simulink model "LeftSteeringWheelButtonsMgr"  (R2022b)
settings: configuration reference "CommonModelConfiguration" (kept outside this file)
undefined symbols (not defined in the file): cc_param_23, cc_param_36, LCFG_ButtonStuck, LCFG_HoldLong, LCFG_HoldShort
settings Model: Creator=sbaumga1  LastModifiedBy=othomso1
settings ConfigSetRef: SourceName=CommonModelConfiguration  SourceLocation=Base Workspace

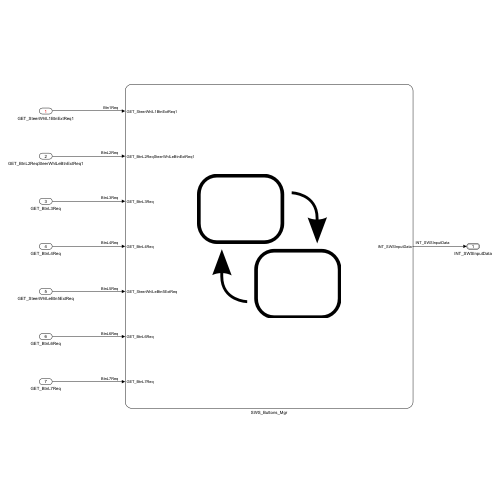
[thumbnail: Simulink's stored preview of the top-level diagram]
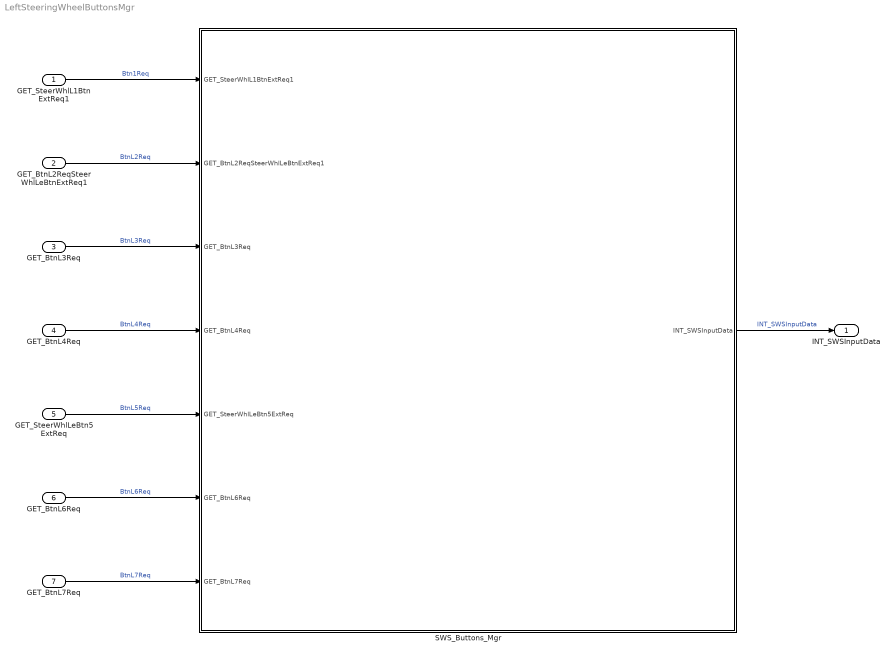
== system LeftSteeringWheelButtonsMgr ==
  GET_SteerWhlL1BtnExtReq1 : Inport  OutDataTypeStr=Enum: PsdNotPsd
  GET_BtnL2ReqSteerWhlLeBtnExtReq1 : Inport  Port=2  OutDataTypeStr=Enum: PsdNotPsd
  GET_BtnL3Req : Inport  Port=3  OutDataTypeStr=Enum: PsdNotPsd
  GET_BtnL4Req : Inport  Port=4  OutDataTypeStr=Enum: PsdNotPsd
  GET_SteerWhlLeBtn5ExtReq : Inport  Port=5  OutDataTypeStr=Enum: PsdNotPsd
  GET_BtnL6Req : Inport  Port=6  OutDataTypeStr=Enum: PsdNotPsd
  GET_BtnL7Req : Inport  Port=7  OutDataTypeStr=Enum: PsdNotPsd
  SWS_Buttons_Mgr : Stateflow chart  TreatAsAtomicUnit=on
  INT_SWSInputData : Outport  OutDataTypeStr=Bus: SWSInputData  BusOutputAsStruct=on
  wires:
  SWS_Buttons_Mgr/1(INT_SWSInputData) -> INT_SWSInputData/1  "INT_SWSInputData"
  GET_BtnL2ReqSteerWhlLeBtnExtReq1/1 -> SWS_Buttons_Mgr/2(GET_BtnL2ReqSteerWhlLeBtnExtReq1)  "BtnL2Req"
  GET_BtnL3Req/1 -> SWS_Buttons_Mgr/3(GET_BtnL3Req)  "BtnL3Req"
  GET_SteerWhlL1BtnExtReq1/1 -> SWS_Buttons_Mgr/1(GET_SteerWhlL1BtnExtReq1)  "Btn1Req"
  GET_BtnL4Req/1 -> SWS_Buttons_Mgr/4(GET_BtnL4Req)  "BtnL4Req"
  GET_SteerWhlLeBtn5ExtReq/1 -> SWS_Buttons_Mgr/5(GET_SteerWhlLeBtn5ExtReq)  "BtnL5Req"
  GET_BtnL6Req/1 -> SWS_Buttons_Mgr/6(GET_BtnL6Req)  "BtnL6Req"
  GET_BtnL7Req/1 -> SWS_Buttons_Mgr/7(GET_BtnL7Req)  "BtnL7Req"

== stateflow chart LeftSteeringWheelButtonsMgr/SWS_Buttons_Mgr ==
  state CARCONFIG_INVALID
  state SYSTEM_OK
    state sws = CheckPsdNotPsd [function]
      (default) -> (junction 458)
      (junction 458) -> (junction 459) [order 1] : [GET_SteerWhlL1BtnExtReq1 == PsdNotPsd.PsdNotPsd_Psd ||...
          | GET_BtnL2ReqSteerWhlLeBtnExtReq1 == PsdNotPsd.PsdNotPsd_Psd ||...
          | GET_BtnL3Req == PsdNotPsd.PsdNotPsd_Psd ||...
          | GET_BtnL4Req == PsdNotPsd.PsdNotPsd_Psd ||...
          | GET_SteerWhlLeBtn5ExtReq == PsdNotPsd.PsdNotPsd_Psd ||...
          | GET_BtnL6Req == PsdNotPsd.PsdNotPsd_Psd ||...
          | GET_BtnL7Req == PsdNotPsd.PsdNotPsd_Psd]
      (junction 458) -> (junction 384) [order 2] : {sws=false;}
      (junction 459) -> (junction 383) : {sws=true;}
      (junction 383) -> (junction 384)
      (junction 384) -> (junction 385)
    state IDLE
      en: INT_SWSInputData.Event = E_SWSEvent.Idle;
      release = false;
      ButtonsReset=false;
    state RELEASE
      en: INT_SWSInputData.Event = E_SWSEvent.Release;
    state PUSHED
      state RUNNING
        entry: ButtonPushed(); btnPush();
        during: ButtonPushed();
        state EVENT
          state PENDING
          state PENDING2
          state HOLDSHORT
            entry: INT_SWSInputData.Event = E_SWSEvent.HoldShort;
          state HOLDLONG
            entry: INT_SWSInputData.Event = E_SWSEvent.HoldLong;
          (default) -> (junction 299)
          (junction 299) -> (junction 488) [order 1] : [INT_SWSInputData.Button == E_SWSButton.BtnL4Req || INT_SWSInputData.Button == E_SWSButton.BtnL5Req]
              | {release = true;}
          (junction 299) -> PENDING [order 2]
          (junction 488) -> PENDING2
          PENDING2 -> HOLDSHORT : [after(LCFG_HoldShort, sec)]
          HOLDSHORT -> HOLDLONG : [after(LCFG_HoldLong, sec)]
        state INVALID_REQUEST
          state IDLE
            en: INT_SWSInputData.Event = E_SWSEvent.Idle;
          state DEACTIVATION
            en: INT_SWSInputData.Event = E_SWSEvent.Deactivation;
          (default) -> SYSTEM_OK.PUSHED.RUNNING.INVALID_REQUEST.IDLE
          SYSTEM_OK.PUSHED.RUNNING.INVALID_REQUEST.IDLE -> DEACTIVATION : [GET_SteerWhlL1BtnExtReq1==PsdNotPsd.PsdNotPsd_Psd]
          DEACTIVATION -> SYSTEM_OK.PUSHED.RUNNING.INVALID_REQUEST.IDLE : [GET_SteerWhlL1BtnExtReq1 ~= PsdNotPsd.PsdNotPsd_Psd]
        state btnPush [function]
          (default) -> (junction 9)
          (junction 9) -> (junction 15) [order 1] : [GET_SteerWhlL1BtnExtReq1 == PsdNotPsd.PsdNotPsd_Psd || GET_BtnL2ReqSteerWhlLeBtnExtReq1 == PsdNotPsd.PsdNotPsd_Psd...
              |  || GET_BtnL3Req == PsdNotPsd.PsdNotPsd_Psd || GET_SteerWhlLeBtn5ExtReq == PsdNotPsd.PsdNotPsd_Psd...
              |  || GET_BtnL6Req == PsdNotPsd.PsdNotPsd_Psd || GET_BtnL7Req == PsdNotPsd.PsdNotPsd_Psd]
          (junction 9) -> (junction 14) [order 2]
          (junction 15) -> (junction 17) : {INT_SWSInputData.Event = E_SWSEvent.Push;}
          (junction 17) -> (junction 14)
        state ButtonPushed [function]
          (default) -> (junction 125) : {ButtonsPressed=0;}
            settings: description=|
                | when two or more buttons on the swsm are pressed at the same time, nothing shall happen until they're all released.
                | exception when button 1 is pressed
          (junction 125) -> (junction 132) [order 1] : [GET_BtnL2ReqSteerWhlLeBtnExtReq1 == PsdNotPsd.PsdNotPsd_Psd]
          (junction 125) -> (junction 414) [order 2]
          (junction 132) -> (junction 130) : {INT_SWSInputData.Button = E_SWSButton.BtnL2Req;
              | ButtonsPressed = ButtonsPressed + 1;}
          (junction 130) -> (junction 414)
          (junction 414) -> (junction 127)
          (junction 127) -> (junction 135) [order 1] : [GET_BtnL3Req == PsdNotPsd.PsdNotPsd_Psd]
          (junction 127) -> (junction 416) [order 2]
          (junction 135) -> (junction 420) : {INT_SWSInputData.Button = E_SWSButton.BtnL3Req;
              | ButtonsPressed = ButtonsPressed + 1;}
          (junction 420) -> (junction 416)
          (junction 416) -> (junction 138)
          (junction 138) -> (junction 143) [order 1] : [GET_BtnL4Req == PsdNotPsd.PsdNotPsd_Psd]
          (junction 138) -> (junction 418) [order 2]
          (junction 143) -> (junction 422) : {INT_SWSInputData.Button = E_SWSButton.BtnL4Req;
              | ButtonsPressed = ButtonsPressed + 1;}
          (junction 422) -> (junction 418)
          (junction 418) -> (junction 139)
          (junction 139) -> (junction 144) [order 1] : [GET_SteerWhlLeBtn5ExtReq == PsdNotPsd.PsdNotPsd_Psd]
          (junction 144) -> (junction 424) : {INT_SWSInputData.Button = E_SWSButton.BtnL5Req;
              | ButtonsPressed = ButtonsPressed + 1;}
          (junction 139) -> (junction 427) [order 2]
          (junction 424) -> (junction 427)
          (junction 427) -> (junction 140)
          (junction 140) -> (junction 145) [order 1] : [GET_BtnL6Req == PsdNotPsd.PsdNotPsd_Psd]
          (junction 140) -> (junction 429) [order 2]
          (junction 145) -> (junction 425) : {INT_SWSInputData.Button = E_SWSButton.BtnL6Req;
              | ButtonsPressed = ButtonsPressed + 1;}
          (junction 425) -> (junction 429)
          (junction 429) -> (junction 146)
          (junction 146) -> (junction 154) [order 1] : [GET_BtnL7Req == PsdNotPsd.PsdNotPsd_Psd]
          (junction 146) -> (junction 431) [order 2]
          (junction 154) -> (junction 426) : {INT_SWSInputData.Button = E_SWSButton.BtnL7Req;
              | ButtonsPressed = ButtonsPressed + 1;}
          (junction 426) -> (junction 431)
          (junction 431) -> (junction 156)
          (junction 156) -> (junction 158) [order 1] : [GET_SteerWhlL1BtnExtReq1 == PsdNotPsd.PsdNotPsd_Psd]
          (junction 156) -> (junction 433) [order 2]
          (junction 158) -> (junction 435) : {INT_SWSInputData.Button = E_SWSButton.BtnL1Req;}
          (junction 435) -> (junction 433)
          (junction 433) -> (junction 440)
          (junction 440) -> (junction 444) [order 1] : [ButtonsPressed>1]
            settings: description=Are more then one button pressed?
          (junction 444) -> (junction 445) : {ButtonsReset=true;}
          (junction 440) -> (junction 442) [order 2]
          (junction 445) -> (junction 442)
          (junction 442) -> (junction 470)
        (default) -> EVENT
        EVENT -> INVALID_REQUEST : [ButtonsReset==1]
      state BUTTON_STUCK
        en: INT_SWSInputData.Event =E_SWSEvent.ButtonStuck;
      (default) -> RUNNING
      RUNNING -> BUTTON_STUCK : [after(LCFG_ButtonStuck,sec)]
    (default) -> SYSTEM_OK.IDLE
    RELEASE -> SYSTEM_OK.IDLE
    PUSHED -> SYSTEM_OK.IDLE [order 2] : [~CheckPsdNotPsd()]
    SYSTEM_OK.IDLE -> PUSHED : [CheckPsdNotPsd()]
    PUSHED -> RELEASE [order 1] : [~CheckPsdNotPsd() &&...
        | release == true]
  (default) -> (junction 480)
  (junction 480) -> CARCONFIG_INVALID [order 2]
  (junction 480) -> SYSTEM_OK [order 1] : [cc_param_23 > 1 || cc_param_36>1]
  data: sws function_output boolean; GET_SteerWhlL1BtnExtReq1 input Enum: PsdNotPsd; INT_SWSInputData output Bus: SWSInputData =0; GET_BtnL2ReqSteerWhlLeBtnExtReq1 input Enum: PsdNotPsd; GET_BtnL3Req input Enum: PsdNotPsd; GET_BtnL4Req input Enum: PsdNotPsd; GET_SteerWhlLeBtn5ExtReq input Enum: PsdNotPsd; GET_BtnL6Req input Enum: PsdNotPsd; GET_BtnL7Req input Enum: PsdNotPsd; LCFG_HoldShort parameter; LCFG_HoldLong parameter; LCFG_ButtonStuck parameter; release local boolean; ButtonsPressed local double; ButtonsReset local boolean =false; cc_param_23 parameter; cc_param_36 parameter
